simulink model "SOCPIControlBenchmarkRealVarL"  (R2019b)
settings: Solver=FixedStepAuto  StartTime=0.0  StopTime=50000  FixedStep=0.01  RelTol=1e-3
values from neighbouring files (symbols this model uses):
  kio = 0.6    [benchmarkPIDStartRealVarL.m]
  kpo = 1    [benchmarkPIDStartRealVarL.m]
  maxKi = 1    [benchmarkPIDStartRealVarL.m]
  maxKp = 1    [benchmarkPIDStartRealVarL.m]
  minKi = 0.01    [benchmarkPIDStartRealVarL.m]
  minKp = 0.01    [benchmarkPIDStartRealVarL.m]
  N = 100    [benchmarkPIDStartRealVarL.m]
  optimPeriod = 300    [benchmarkPIDStartRealVarL.m]
  OVLim = 2    [benchmarkPIDStartRealVarL.m]
  refAmplitude = 50    [benchmarkPIDStartRealVarL.m]
  refSignalPeriod = optimPeriod    (= 300)    [benchmarkPIDStartRealVarL.m]
  resetThreshold = 0.1    [benchmarkPIDStartRealVarL.m]
undefined symbols (not defined in the file or in its folder): FORandGCNM, sigbuilder_block
libraries: dspmathops x3, simulink x1
(part 4 of 4)

== matlab function SOCPIControlBenchmarkRealVarL/Original NM1/Original NM Control/Original NM ==
  data: f input; y output size=2; x input; NM_state_val output
function [y, NM_state_val] = fcn(f, x)
% Acknowledgement goes to Mathworks' FMINSEARCH, borrowed some code snippets
% persistent count

persistent NM_state         %Integer definition for states, since enum is not supported
persistent Full_eval_count
persistent usual_delta      %5 percent deltas for non-zero terms
persistent zero_term_delta  %Even smaller delta for zero elements of x
persistent v fv v_r v_e v_m f_r v_c

n = 2;      %Input dimension - needs to be defined as a constant to keep Simulink port width inheretence happy
np1 = n+1;

n_r = 1/n;  %Calculate reciprocal at compilation time for mean calculation

%Simplex update coefficients %Can be a function of dimension see Han2010
alpha = 1;
beta = 2;
gamma = 0.5;
delta = 0.5;

%Adaptive simplex search coefficients: Han2010
% alpha = 1;
% beta = 1 + 2*n_r;
% gamma = 0.75 - 0.5*n_r;
% delta = 1 - n_r;
% 
% alpha = 0.25;
% beta = 1 + 2*n_r;
% gamma = 0.75 - 0.5*n_r;
% delta = 1 - n_r;


%NM_state:  
    %0 - Initial   (Initialize vertices)+++++
    %1 - FVE: Full vertex evaluation (with insertion sort after each
    %evaluation)++++++
    %2 - Insertion Sort (After Reflection, Expansion or Contraction Steps)
    %3 - Reflection Entry
    %4 - Reflection Evaluate+++++++++++++++++
    %5 - Expansion++++++++++++
    %6 - Outside Contraction++++++++++++
    %7 - Inside Contraction++++++++++++++++
    %(8) - Shrink (Implicit on contraction outcome)

%Full_eval_count:
    %Number of initial vertices evaluated


xin = x(:);         %Force xin to be a column vector

    if isempty(NM_state)
        v = zeros(n,np1);   %Initialize n+1 vertices for simplex
        fv = zeros(1,np1);  %function values at the vertices
        fv(1)=f;%initialize in the initial condition the first vertex
        
        
        v_m = v(:,1);       %0 vector centroid
        v_r = v_m;          %0 vector reflection   
        v_e = v_m;          %0 vector expansion
        v_c = v_m;          %0 vector contraction
        f_r = 0;          %0 vector

        usual_delta = 0.05;
        zero_term_delta = 0.00025;
        NM_state = 0;          %Initial state
        Full_eval_count = 1;   %No vertices evaulated, yet

        v(:,1) = xin;
        for j=1:n
            vt = xin;
            if vt(j) ~= 0
                vt(j) = (1 + usual_delta)*vt(j);
            else
                vt(j) = zero_term_delta;
            end
            v(:, j+1) = vt;
        end
        v;
    end
           
    switch NM_state  
        case 0 %Vertices has just been initialized
          y = v(:, Full_eval_count); %Write out first vertex for evaluation
          NM_state = 1;
          
        case 1 %Full vertex evaluation  and reflection on the final part
            fv(Full_eval_count) = f;  %Read evaluated function value
            
            %sort values
            j = Full_eval_count;  %New value came in, insert it into sorted list
            while ( (j>1) && (fv(j-1)>fv(j)) ) %Sort ascending
               temp = fv(j-1);
               fv(j-1) = fv(j);
               fv(j) = temp;
               temp = v(:, j-1);
               v(:, j-1) = v(:, j); %Also sort corresponding (evaluated) vertices 
               v(:, j) = temp;
               j = j-1;
            end
             
            Full_eval_count = Full_eval_count + 1;            
            if (Full_eval_count <= (np1))
                y = v(:, Full_eval_count);                
            else
                Full_eval_count = Full_eval_count - 1; 
                %NM_state = 3;   %Full vertex evaluation complete -> Reflection 
                v_sum = xin*0;  %Initialize sum for mean calculation

                for i=1:n
                    v_sum = v_sum + v(:, i);
                end

                v_m = v_sum*n_r; %Centroid (mean point of the two best points)
                v_r  = v_m*(1+alpha) - alpha*v(:, end);   %reflection vertex calculation
                y  = v_r;       %set as next output the reflection vertex
                NM_state = 4;   %jump to Reflection Evaluate
            end
            
%         case 2 %Insertion Sort                        
%                 j = Full_eval_count;  %New value came in, insert it into list
%                    while ( (j>1) && (fv(j-1)>fv(j)) ) %Sort ascending
%                        temp = fv(j-1);
%                        fv(j-1) = fv(j);
%                        fv(j) = temp;
%                        temp = v(:, j-1);
%                        v(:, j-1) = v(:, j); %Also sort corresponding (evaluated) vertices 
%                        v(:, j) = temp;
%                        j = j-1;
%                    end
%                 NM_state = 3;   %Reflection 
            
%         case 3 %Reflection Entry
%                 v_sum = xin*0;  %Initialize sum for mean calculation
% 
%                 for i=1:n
%                     v_sum = v_sum + v(:, i);
%                 end
% 
%                 v_m = v_sum*n_r; %Centroid
%                 v_r  = v_m*(1+alpha) - alpha*v(:, np1);
%                 y  = v_r;
%                 NM_state = 4;   %Reflection Evaluate

        case 4 %Reflection Evaluation (after reflection is calculated and applied on the previous step)
            f_r = f;
%             if ( (f_r<fv(:, 1)) && (f_r>fv(:, n)) )  

            if ( (f_r>fv(:, 1)) && (f_r<fv(:, n)) )  
                v(:, np1) = v_r;
                fv(np1) = f_r;
                %NM_state = 2;
                j = Full_eval_count;  %New value came in, insert it into list
                while ( (j>1) && (fv(j-1)>fv(j)) ) %Sort ascending
                   temp = fv(j-1);
                   fv(j-1) = fv(j);
                   fv(j) = temp;
                   temp = v(:, j-1);
                   v(:, j-1) = v(:, j); %Also sort corresponding (evaluated) vertices 
                   v(:, j) = temp;
                   j = j-1;
                end
                %%NM_state = 3;   %Reflection 

                v_sum = xin*0;  %Initialize sum for mean calculation

                for i=1:n
                    v_sum = v_sum + v(:, i);
                end

                v_m = v_sum*n_r; %Centroid
                v_r  = v_m*(1+alpha) - alpha*v(:, np1);
                y  = v_r;
                NM_state = 4;    %Reflection Evaluate
            elseif (f_r<fv(:, 1))
                v_e  = v_m*(1-beta) + beta*v_r; 
                y  = v_e;
                NM_state = 5;    %Expansion
            else
                if ( (f_r>=fv(n)) && (f_r<fv(np1)) ) 
                    v_c  = v_m*(1-gamma) + gamma*v_r; 
                    NM_state = 6; %Outside Contraction
                elseif (f_r>=fv(np1))  
                    v_c  = v_m*(1+gamma) - gamma*v_r; 
                    NM_state = 7; %Inside Contraction
                end
                y = v_c;
            end
            
        case 5 %Expansion
            f_e = f;
            if (f_e<f_r)
                v(:, end) = v_e;
                fv(end) = f_e;
                %NM_state = 2;
                    j = Full_eval_count;  %New value came in, insert it into list
                   while ( (j>1) && (fv(j-1)>fv(j)) ) %Sort ascending
                       temp = fv(j-1);
                       fv(j-1) = fv(j);
                       fv(j) = temp;
                       temp = v(:, j-1);
                       v(:, j-1) = v(:, j); %Also sort corresponding (evaluated) vertices 
                       v(:, j) = temp;
                       j = j-1;
                   end
                %%NM_state = 3;   %Reflection 

                v_sum = xin*0;  %Initialize sum for mean calculation

                for i=1:n
                    v_sum = v_sum + v(:, i);
                end

                v_m = v_sum*n_r; %Centroid
                v_r  = v_m*(1+alpha) - alpha*v(:, np1);
                y  = v_r;
                NM_state = 4;   %Reflection Evaluate
             else
                v(:, np1) = v_r;
                fv(np1) = f_r;
                %NM_state = 2;
                j = Full_eval_count;  %New value came in, insert it into list
               while ( (j>1) && (fv(j-1)>fv(j)) ) %Sort ascending
                   temp = fv(j-1);
                   fv(j-1) = fv(j);
                   fv(j) = temp;
                   temp = v(:, j-1);
                   v(:, j-1) = v(:, j); %Also sort corresponding (evaluated) vertices 
                   v(:, j) = temp;
                   j = j-1;
               end
               
               %%NM_state = 3;   %Reflection 

                v_sum = xin*0;  %Initialize sum for mean calculation

                for i=1:n
                    v_sum = v_sum + v(:, i);
                end

                v_m = v_sum*n_r; %Centroid
                v_r  = v_m*(1+alpha) - alpha*v(:, np1);
                y  = v_r;
                NM_state = 4;   %Reflection Evaluate
            end
            
       case 6 %Contraction
           f_c = f;
           if (f_c<f_r)
               v(:, np1) = v_c;
               fv(np1) = f_c;
               %NM_state = 2;
               j = Full_eval_count;  %New value came in, insert it into list
               while ( (j>1) && (fv(j-1)>fv(j)) ) %Sort ascending
                   temp = fv(j-1);
                   fv(j-1) = fv(j);
                   fv(j) = temp;
                   temp = v(:, j-1);
                   v(:, j-1) = v(:, j); %Also sort corresponding (evaluated) vertices 
                   v(:, j) = temp;
                   j = j-1;
               end
                %%NM_state = 3;   %Reflection 

                v_sum = xin*0;  %Initialize sum for mean calculation

                for i=1:n
                    v_sum = v_sum + v(:, i);
                end

                v_m = v_sum*n_r; %Centroid
                v_r  = v_m*(1+alpha) - alpha*v(:, np1);
                y  = v_r;
                NM_state = 4;   %Reflection Evaluate
           else
               for j=2:n+1   %Shrink
                 v(:,j) = v(:,1)*(1-delta) + delta*v(:,j);
               end
               y = v(:, 2);   %Start with evaluation
               Full_eval_count = 2; 
               NM_state = 1; %Full vertex evaluation after shrink
           end
        case 7
            f_c = f;
               if (f_c<fv(np1))
                   v(:, np1) = v_c;
                   fv(np1) = f_c;
                   %NM_state = 2;
                    j = Full_eval_count;  %New value came in, insert it into list
                    while ( (j>1) && (fv(j-1)>fv(j)) ) %Sort ascending
                       temp = fv(j-1);
                       fv(j-1) = fv(j);
                       fv(j) = temp;
                       temp = v(:, j-1);
                       v(:, j-1) = v(:, j); %Also sort corresponding (evaluated) vertices 
                       v(:, j) = temp;
                       j = j-1;
                    end
                    %%NM_state = 3;   %Reflection 

                    v_sum = xin*0;  %Initialize sum for mean calculation

                    for i=1:n
                        v_sum = v_sum + v(:, i);
                    end

                    v_m = v_sum*n_r; %Centroid
                    v_r  = v_m*(1+alpha) - alpha*v(:, np1);
                    y  = v_r;
                    NM_state = 4;   %Reflection Evaluate
               else
                   for j=2:n+1 %Shrink
                     v(:,j) = v(:,1)*(1-delta) + delta*v(:,j);
                   end
                   y = v(:,2);   %Start with evaluation
                   Full_eval_count = 2; 
                   NM_state = 1; %Full vertex evaluation after shrink  
               end     
        otherwise
        y = v(:,1);
     end %End switch NM_states     
     NM_state_val = NM_state;
end %End of function

== matlab function SOCPIControlBenchmarkRealVarL/Original NM1/Original NM Control/Original NM2 ==
  settings: updateMethod=DISCRETE
  data: f input; y output size=2; x input; NM_state_val output; YY output
function [y, NM_state_val, YY] = fcn(f, x)
% Acknowledgement goes to Mathworks' FMINSEARCH, borrowed some code snippets
% persistent count

persistent NM_state         %Integer definition for states, since enum is not supported
persistent Full_eval_count
persistent usual_delta      %5 percent deltas for non-zero terms
persistent zero_term_delta  %Even smaller delta for zero elements of x
persistent v fv v_r v_e v_m f_r v_c

n = 2;      %Input dimension - needs to be defined as a constant to keep Simulink port width inheretence happy
np1 = n+1;

n_r = 1/n;  %Calculate reciprocal at compilation time for mean calculation

%Simplex update coefficients %Can be a function of dimension see Han2010
alpha = 1;
beta = 2;
gamma = 0.5;
delta = 0.5;

%Adaptive simplex search coefficients: Han2010
% alpha = 1;
% beta = 1 + 2*n_r;
% gamma = 0.75 - 0.5*n_r;
% delta = 1 - n_r;
% % 
% alpha = 1;           %reflection
% beta = 1 + 2*n_r;       %expansion
% gamma = 0.75 - 0.5*n_r; %contraction
% delta = 1 - n_r;        %shrinking


%NM_state:  
    %0 - Initial   (Initialize vertices)+++++
    %1 - FVE: Full vertex evaluation (with insertion sort after each
    %evaluation)++++++
    %2 - Insertion Sort (After Reflection, Expansion or Contraction Steps)
    %3 - Reflection Entry
    %4 - Reflection Evaluate+++++++++++++++++
    %5 - Expansion++++++++++++
    %6 - Outside Contraction++++++++++++
    %7 - Inside Contraction++++++++++++++++
    %(8) - Shrink (Implicit on contraction outcome)

%Full_eval_count:
    %Number of initial vertices evaluated


xin = x(:);         %Force xin to be a column vector

    if isempty(NM_state)
        v = zeros(n,np1);   %Initialize n+1 vertices for simplex
        fv = zeros(1,np1);  %function values at the vertices
        fv(1)=f;%initialize in the initial condition the first vertex
        
        
        v_m = v(:,1);       %0 vector centroid
        v_r = v_m;          %0 vector reflection   
        v_e = v_m;          %0 vector expansion
        v_c = v_m;          %0 vector contraction
        f_r = 0;          %0 vector

%         usual_delta = 0.05;
        usual_delta = 1;
        zero_term_delta = 0.00025;
        NM_state = 0;          %Initial state
        Full_eval_count = 1;   %No vertices evaulated, yet

        v(:,1) = xin;
        for j=1:n
            vt = xin;
            if vt(j) ~= 0
                vt(j) = (1 + usual_delta)*vt(j);
            else
                vt(j) = zero_term_delta;
            end
            v(:, j+1) = vt;
        end
        v;
    end
           
    switch NM_state  
        case 0 %Vertices has just been initialized
          y = v(:, Full_eval_count); %Write out first vertex for evaluation
          NM_state = 1;
          
        case 1 %Full vertex evaluation  and reflection on the final part
            fv(Full_eval_count) = f;  %Read evaluated function value
            
            %sort values
            j = Full_eval_count;  %New value came in, insert it into sorted list
            while ( (j>1) && (fv(j-1)>fv(j)) ) %Sort ascending
               temp = fv(j-1);
               fv(j-1) = fv(j);
               fv(j) = temp;
               temp = v(:, j-1);
               v(:, j-1) = v(:, j); %Also sort corresponding (evaluated) vertices 
               v(:, j) = temp;
               j = j-1;
            end
             
            Full_eval_count = Full_eval_count + 1;            
            if (Full_eval_count <= (np1))
                y = v(:, Full_eval_count);                
            else
                Full_eval_count = Full_eval_count - 1; 
                %NM_state = 3;   %Full vertex evaluation complete -> Reflection 
                v_sum = xin*0;  %Initialize sum for mean calculation

                for i=1:n
                    v_sum = v_sum + v(:, i);
                end

                v_m = v_sum*n_r; %Centroid (mean point of the two best points)
                v_r  = v_m*(1+alpha) - alpha*v(:, end);   %reflection vertex calculation
                y  = v_r;       %set as next output the reflection vertex
                NM_state = 4;   %jump to Reflection Evaluate
            end
            
%         case 2 %Insertion Sort                        
%                 j = Full_eval_count;  %New value came in, insert it into list
%                    while ( (j>1) && (fv(j-1)>fv(j)) ) %Sort ascending
%                        temp = fv(j-1);
%                        fv(j-1) = fv(j);
%                        fv(j) = temp;
%                        temp = v(:, j-1);
%                        v(:, j-1) = v(:, j); %Also sort corresponding (evaluated) vertices 
%                        v(:, j) = temp;
%                        j = j-1;
%                    end
%                 NM_state = 3;   %Reflection 
            
%         case 3 %Reflection Entry
%                 v_sum = xin*0;  %Initialize sum for mean calculation
% 
%                 for i=1:n
%                     v_sum = v_sum + v(:, i);
%                 end
% 
%                 v_m = v_sum*n_r; %Centroid
%                 v_r  = v_m*(1+alpha) - alpha*v(:, np1);
%                 y  = v_r;
%                 NM_state = 4;   %Reflection Evaluate

        case 4 %Reflection Evaluation (after reflection is calculated and applied on the previous step)
            f_r = f;
%             if ( (f_r<fv(:, 1)) && (f_r>fv(:, n)) )  

            if ( (f_r>fv(:, 1)) && (f_r<fv(:, n)) )  
                v(:, np1) = v_r;
                fv(np1) = f_r;
                %NM_state = 2;
                j = Full_eval_count;  %New value came in, insert it into list
                while ( (j>1) && (fv(j-1)>fv(j)) ) %Sort ascending
                   temp = fv(j-1);
                   fv(j-1) = fv(j);
                   fv(j) = temp;
                   temp = v(:, j-1);
                   v(:, j-1) = v(:, j); %Also sort corresponding (evaluated) vertices 
                   v(:, j) = temp;
                   j = j-1;
                end
                %%NM_state = 3;   %Reflection 

                v_sum = xin*0;  %Initialize sum for mean calculation

                for i=1:n
                    v_sum = v_sum + v(:, i);
                end

                v_m = v_sum*n_r; %Centroid
                v_r  = v_m*(1+alpha) - alpha*v(:, np1);
                y  = v_r;
                NM_state = 4;    %Reflection Evaluate
            elseif (f_r<fv(:, 1))
                v_e  = v_m*(1-beta) + beta*v_r; 
                y  = v_e;
                NM_state = 5;    %Expansion
            else
                if ( (f_r>=fv(n)) && (f_r<fv(np1)) ) 
                    v_c  = v_m*(1-gamma) + gamma*v_r; 
                    NM_state = 6; %Outside Contraction
                elseif (f_r>=fv(np1))  
                    v_c  = v_m*(1+gamma) - gamma*v_r; 
                    NM_state = 7; %Inside Contraction
                end
                y = v_c;
            end
            
        case 5 %Expansion
            f_e = f;
            if (f_e<f_r)
                v(:, end) = v_e;
                fv(end) = f_e;
                %NM_state = 2;
                    j = Full_eval_count;  %New value came in, insert it into list
                   while ( (j>1) && (fv(j-1)>fv(j)) ) %Sort ascending
                       temp = fv(j-1);
                       fv(j-1) = fv(j);
                       fv(j) = temp;
                       temp = v(:, j-1);
                       v(:, j-1) = v(:, j); %Also sort corresponding (evaluated) vertices 
                       v(:, j) = temp;
                       j = j-1;
                   end
                %%NM_state = 3;   %Reflection 

                v_sum = xin*0;  %Initialize sum for mean calculation

                for i=1:n
                    v_sum = v_sum + v(:, i);
                end

                v_m = v_sum*n_r; %Centroid
                v_r  = v_m*(1+alpha) - alpha*v(:, np1);
                y  = v_r;
                NM_state = 4;   %Reflection Evaluate
             else
                v(:, np1) = v_r;
                fv(np1) = f_r;
                %NM_state = 2;
                j = Full_eval_count;  %New value came in, insert it into list
               while ( (j>1) && (fv(j-1)>fv(j)) ) %Sort ascending
                   temp = fv(j-1);
                   fv(j-1) = fv(j);
                   fv(j) = temp;
                   temp = v(:, j-1);
                   v(:, j-1) = v(:, j); %Also sort corresponding (evaluated) vertices 
                   v(:, j) = temp;
                   j = j-1;
               end
               
               %%NM_state = 3;   %Reflection 

                v_sum = xin*0;  %Initialize sum for mean calculation

                for i=1:n
                    v_sum = v_sum + v(:, i);
                end

                v_m = v_sum*n_r; %Centroid
                v_r  = v_m*(1+alpha) - alpha*v(:, np1);
                y  = v_r;
                NM_state = 4;   %Reflection Evaluate
            end
            
       case 6 %Contraction
           f_c = f;
           if (f_c<f_r)
               v(:, np1) = v_c;
               fv(np1) = f_c;
               %NM_state = 2;
               j = Full_eval_count;  %New value came in, insert it into list
               while ( (j>1) && (fv(j-1)>fv(j)) ) %Sort ascending
                   temp = fv(j-1);
                   fv(j-1) = fv(j);
                   fv(j) = temp;
                   temp = v(:, j-1);
                   v(:, j-1) = v(:, j); %Also sort corresponding (evaluated) vertices 
                   v(:, j) = temp;
                   j = j-1;
               end
                %%NM_state = 3;   %Reflection 

                v_sum = xin*0;  %Initialize sum for mean calculation

                for i=1:n
                    v_sum = v_sum + v(:, i);
                end

                v_m = v_sum*n_r; %Centroid
                v_r  = v_m*(1+alpha) - alpha*v(:, np1);
                y  = v_r;
                NM_state = 4;   %Reflection Evaluate
           else
               for j=2:n+1   %Shrink
                 v(:,j) = v(:,1)*(1-delta) + delta*v(:,j);
               end
               y = v(:, 2);   %Start with evaluation
               Full_eval_count = 2; 
               NM_state = 1; %Full vertex evaluation after shrink
           end
        case 7
            f_c = f;
               if (f_c<fv(np1))
                   v(:, np1) = v_c;
                   fv(np1) = f_c;
                   %NM_state = 2;
                    j = Full_eval_count;  %New value came in, insert it into list
                    while ( (j>1) && (fv(j-1)>fv(j)) ) %Sort ascending
                       temp = fv(j-1);
                       fv(j-1) = fv(j);
                       fv(j) = temp;
                       temp = v(:, j-1);
                       v(:, j-1) = v(:, j); %Also sort corresponding (evaluated) vertices 
                       v(:, j) = temp;
                       j = j-1;
                    end
                    %%NM_state = 3;   %Reflection 

                    v_sum = xin*0;  %Initialize sum for mean calculation

                    for i=1:n
                        v_sum = v_sum + v(:, i);
                    end

                    v_m = v_sum*n_r; %Centroid
                    v_r  = v_m*(1+alpha) - alpha*v(:, np1);
                    y  = v_r;
                    NM_state = 4;   %Reflection Evaluate
               else
                   for j=2:n+1 %Shrink
                     v(:,j) = v(:,1)*(1-delta) + delta*v(:,j);
                   end
                   y = v(:,2);   %Start with evaluation
                   Full_eval_count = 2; 
                   NM_state = 1; %Full vertex evaluation after shrink  
               end     
        otherwise
        y = v(:,1);
       
     end %End switch NM_states     
     NM_state_val = NM_state;
      YY=v;
end %End of function

== matlab function SOCPIControlBenchmarkRealVarL/Original NM1/determinant simplex aware ==
  data: u input; vv1 output; v12 output; v21 output; v1n output; v2n output
function [vv1,v12,v21,v1n,v2n]= fcn(u)
    vv1=u;
    v12=abs(det(vv1(:,2:3)));
    vaux=[vv1(:,1)-vv1(:,2)  vv1(:,1)-vv1(:,3)  ];
    v21=abs(det(vaux));
    
    v1n=norm(vv1(:,2),2);
    v2n=norm(vv1(:,3),2);
    
    
end
